simulink model "pid_suspension"  (R2025a)
settings: Solver=ode23s  StartTime=0.0  StopTime=T_sim  RelTol=1e-3
undefined symbols (not defined in the file): Kd, Ki, Kp, ks, kt, ms, mus, zs_static, zus_static
libraries: slpidlib x1
settings Model: Creator=Anderson  LastModifiedBy=Anderson
settings DataIOCC: SaveFormat=StructureWithTime

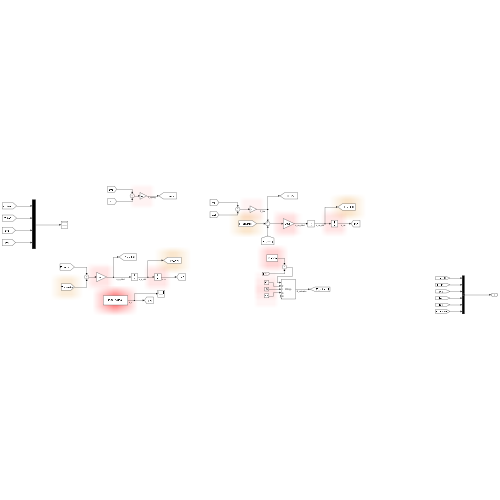
[thumbnail: Simulink's stored preview of the top-level diagram]
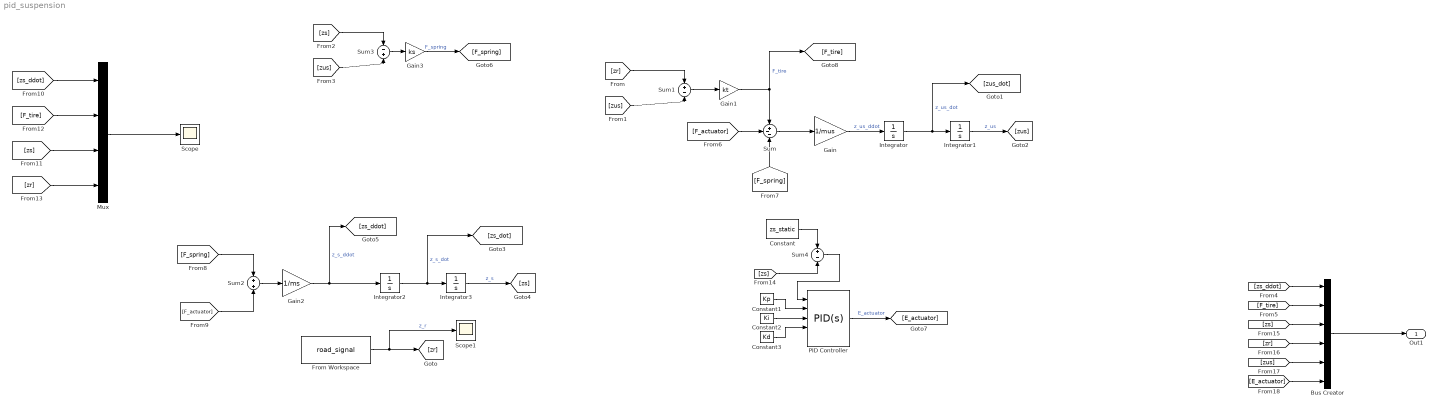
== system pid_suspension ==
  Bus Creator : BusCreator  Inputs=6
  Constant : Constant  Value=zs_static
  Constant1 : Constant  Value=Kp
  Constant2 : Constant  Value=Ki
  Constant3 : Constant  Value=Kd
  From Workspace : FromWorkspace  VariableName=road_signal
  Gain : Gain  Gain=1/mus
  Gain1 : Gain  Gain=kt
  Gain2 : Gain  Gain=1/ms
  Gain3 : Gain  Gain=ks
  Integrator : Integrator
  Integrator1 : Integrator  InitialCondition=zus_static
  Integrator2 : Integrator
  Integrator3 : Integrator  InitialCondition=zs_static
  Mux : Mux
  PID Controller : slpidlib/PID Controller  Controller=PID  Form=Parallel  TimeDomain=Continuous-time  UseExternalTs=off  SampleTime=-1  IntegratorMethod=Forward Euler  FilterMethod=Forward Euler  ControllerParametersSource=external  P=1  I=1  UseKiTs=off  D=0  UseExternalDerivativeSource=off  N=100  UseFilter=on  TunerSelectOption=Transfer Function Based (PID Tuner App)  InitialConditionSource=internal  InitialConditionForIntegrator=0  InitialConditionForFilter=0  DifferentiatorICPrevScaledInput=0  ExternalReset=none  TrackingMode=off  Kt=1  LimitOutput=off  SatLimitsSource=internal  UpperSaturationLimit=inf  LowerSaturationLimit=-inf  LinearizeAsGain=on  AntiWindupMode=none  Kb=1  LimitIntegrator=off  UpperIntegratorSaturationLimit=inf  LowerIntegratorSaturationLimit=-inf  POutMin=[]  POutMax=[]  IOutMin=[]  IOutMax=[]  DOutMin=[]  DOutMax=[]  NOutMin=[]  NOutMax=[]  SumOutMin=[]  SumOutMax=[]  SaturationOutMin=[]  SaturationOutMax=[]  PParamMin=[]  PParamMax=[]  IParamMin=[]  IParamMax=[]  DParamMin=[]  DParamMax=[]  NParamMin=[]  NParamMax=[]  KbParamMin=[]  KbParamMax=[]  KtParamMin=[]  KtParamMax=[]  KbOutMin=[]  KbOutMax=[]  KtOutMin=[]  KtOutMax=[]  IntegratorOutMin=[]  IntegratorOutMax=[]  FilterOutMin=[]  FilterOutMax=[]  SumI1OutMin=[]  SumI1OutMax=[]  SumI2OutMin=[]  SumI2OutMax=[]  SumI3OutMin=[]  SumI3OutMax=[]  SumI4OutMin=[]  SumI4OutMax=[]  SumDOutMin=[]  SumDOutMax=[]  DifferentiatorOutMin=[]  DifferentiatorOutMax=[]  FilterDiffOutCoefMin=[]  FilterDiffOutCoefMax=[]  ReciprocalOutMin=[]  ReciprocalOutMax=[]  SumDenOutMin=[]  SumDenOutMax=[]  SumNumOutMin=[]  SumNumOutMax=[]  DivideOutMin=[]  DivideOutMax=[]  UdiffTsProdOutMin=[]  UdiffTsProdOutMax=[]  NTsProdOutMin=[]  NTsProdOutMax=[]  UintegralTsProdOutMin=[]  UintegralTsProdOutMax=[]  UngainTsProdOutMin=[]  UngainTsProdOutMax=[]  ClampingZeroOutDataTypeStr=Inherit: Inherit via back propagation  ClampingZeroOutMin=[]  ClampingZeroOutMax=[]  FilterDenConstantOutDataTypeStr=Inherit: Inherit via back propagation  FilterDenConstantOutMin=[]  FilterDenConstantOutMax=[]  PCopyOutDataTypeStr=Inherit: Inherit via back propagation  PCopyOutMin=[]  PCopyOutMax=[]  NCopyOutDataTypeStr=Inherit: Inherit via back propagation  NCopyOutMin=[]  NCopyOutMax=[]  IntegratorContinuousStateAttributes=''  IntegratorStateMustResolveToSignalObject=off  IntegratorRTWStateStorageClass=Auto  FilterContinuousStateAttributes=''  FilterStateMustResolveToSignalObject=off  FilterRTWStateStorageClass=Auto  ParallelPVariant=ExternalParameters  IdealPVariant=Disabled  IVariant=ExternalParameters  DVariant=ExternalParameters  IntegratorVariant=Continuous  SatVariant=Disabled  AWVariant=Passthrough  PCopyVariant=Disabled  TRVariant=Disabled  FdbkBlocksVariant=Forward  IdealPFdbkVariant=Disabled  SatFdbkVariant=Disabled  DerivativeFilterVariant=ContFilter  NVariant=ExternalParameters  NCopyVariant=Disabled  FilterICVariant=InternalICsFilter  IntegratorICVariant=InternalICs  ExternalResetVariant=Disabled  TRSumVariant=Passthrough  SumFdbkVariant=Disabled  SumVariant=Sum_PID  TsampFilterVariant=InternalTs  TsampNgainVariant=Passthrough  TsampIntegralVariant=Disabled_SignalSpec  ExternalSaturationOutDataTypeStr=Inherit: Same as second input  DerivativeSourceVariant=ErrorSignal  PreIntVariant=InternalPreInt
  Scope : Scope
      settings: ActiveDisplayYMinimum=-6868.1819363859859  ActiveDisplayYMaximum=4567.23132626511
  Scope1 : Scope
      settings: ActiveDisplayYMinimum=-0.012493378905301503  ActiveDisplayYMaximum=0.11244041014771355
  Sum : Sum  Inputs=+--
  Sum1 : Sum  Inputs=+-
  Sum2 : Sum
  Sum3 : Sum  Inputs=-+
  Sum4 : Sum  Inputs=+-
  Out1 : Outport
  wires:
  From Workspace/1 -> [zr], Scope1/1  "z_r"
  Integrator/1 -> [zus_dot], Integrator1/1  "z_us_dot"
  Gain/1 -> Integrator/1  "z_us_ddot​"
  Integrator1/1 -> [zus]  "z_us"
  Sum/1 -> Gain/1
  [zr] -> Sum1/1
  [zus] -> Sum1/2
  Sum1/1 -> Gain1/1
  Gain1/1 -> Sum/1, [F_tire]  "F_tire"
  Gain2/1 -> [zs_ddot], Integrator2/1  "z_s_ddot"
  Integrator2/1 -> [zs_dot], Integrator3/1  "z_s_dot"
  Integrator3/1 -> [zs]  "z_s"
  Sum2/1 -> Gain2/1
  [zs] -> Sum3/1
  [zus] -> Sum3/2
  Sum3/1 -> Gain3/1
  Gain3/1 -> [F_spring]  "F_spring"
  [F_spring] -> Sum/3
  [F_actuator] -> Sum/2
  [F_spring] -> Sum2/1
  [F_actuator] -> Sum2/2
  [zs_ddot] -> Mux/1
  [F_tire] -> Mux/2
  [zs] -> Mux/3
  [zr] -> Mux/4
  Mux/1 -> Scope/1
  Constant/1 -> Sum4/1
  [zs] -> Sum4/2
  Constant1/1 -> PID Controller/2
  Constant2/1 -> PID Controller/3
  Constant3/1 -> PID Controller/4
  Sum4/1 -> PID Controller/1
  PID Controller/1 -> [E_actuator]  "E_actuator"
  [zs_ddot] -> Bus Creator/1
  [F_tire] -> Bus Creator/2
  [zs] -> Bus Creator/3
  [zr] -> Bus Creator/4
  [zus] -> Bus Creator/5
  [E_actuator] -> Bus Creator/6
  Bus Creator/1 -> Out1/1
